simulink model "EJ10_6"  (R2022a)
settings: Solver=FixedStepAuto  StartTime=0.0  StopTime=4  FixedStep=0.001  RelTol=1e-3
settings Model: Creator=Idael  LastModifiedBy=benja

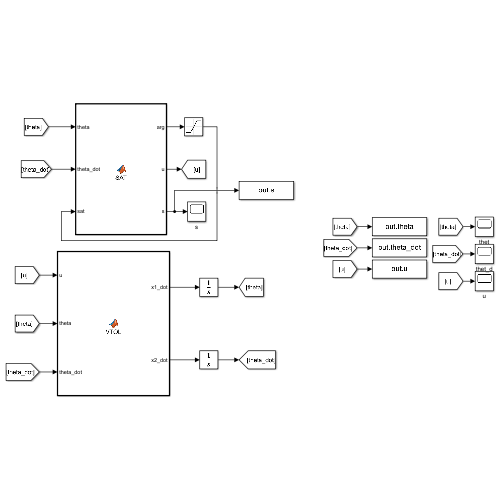
[thumbnail: Simulink's stored preview of the top-level diagram]
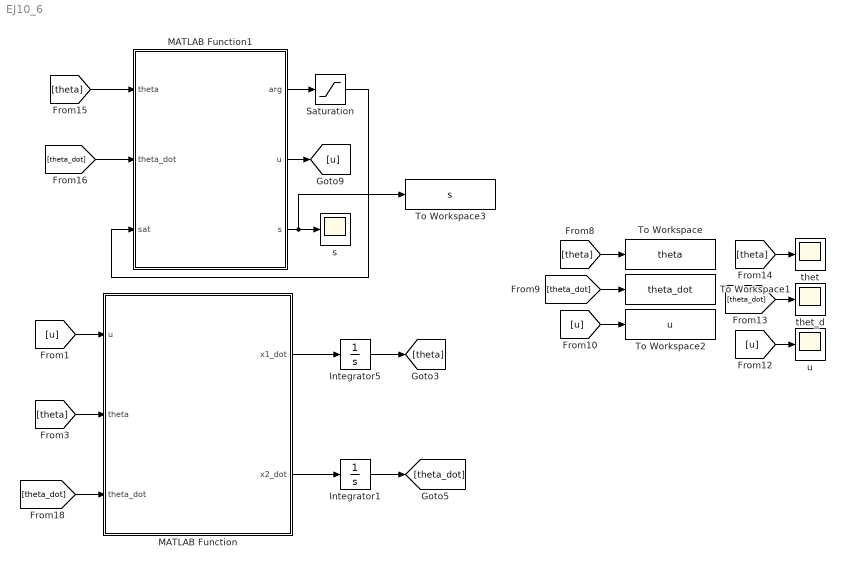
== system EJ10_6 ==
  Integrator1 : Integrator
  Integrator5 : Integrator
  MATLAB Function : MATLAB Function  TreatAsAtomicUnit=on
  MATLAB Function1 : MATLAB Function  TreatAsAtomicUnit=on
  Saturation : Saturate  UpperLimit=1  LowerLimit=-1
  To Workspace : ToWorkspace  VariableName=theta  SampleTime=-1
  To Workspace1 : ToWorkspace  VariableName=theta_dot  SampleTime=-1
  To Workspace2 : ToWorkspace  VariableName=u  SampleTime=-1
  To Workspace3 : ToWorkspace  VariableName=s  SampleTime=-1
  s : Scope
  thet : Scope
  thet_d : Scope
  u : Scope
  wires:
  [theta] -> To Workspace/1
  [theta_dot] -> To Workspace1/1
  [u] -> To Workspace2/1
  MATLAB Function/1(x1_dot) -> Integrator5/1
  MATLAB Function/2(x2_dot) -> Integrator1/1
  [u] -> u/1
  [theta_dot] -> thet_d/1
  [theta] -> thet/1
  Integrator5/1 -> [theta]
  Integrator1/1 -> [theta_dot]
  [theta] -> MATLAB Function1/1(theta)
  [theta_dot] -> MATLAB Function/3(theta_dot)
  MATLAB Function1/2(u) -> [u]
  [u] -> MATLAB Function/1(u)
  [theta_dot] -> MATLAB Function1/2(theta_dot)
  MATLAB Function1/1(arg) -> Saturation/1
  Saturation/1 -> MATLAB Function1/3(sat)
  [theta] -> MATLAB Function/2(theta)
  MATLAB Function1/3(s) -> To Workspace3/1, s/1

== matlab function EJ10_6/MATLAB Function1 ==
  data: theta input; theta_dot input; arg output; sat input; u output; s output
function [arg,u,s]  = SAT(theta,theta_dot,sat)
  mu=0.1;
  s=theta-(pi/2)+theta_dot;
  arg=s/mu;
%   u=-(2.5+2*abs(theta_dot))*sat;
  u=-(2.5+2*abs(theta_dot))*(s/0.1);
end

== matlab function EJ10_6/MATLAB Function ==
  data: u input; theta input; theta_dot input; x1_dot output; x2_dot output
function [x1_dot,x2_dot] = VTOL(u,theta,theta_dot)
b0 = 0.01;
c = 0.5;

x1_dot=theta_dot;
x2_dot=-sin(theta)-b0*theta_dot+c*u;
end
